simulink model "DAB"  (R2018b)
settings: Solver=ode23t  StartTime=0.0  StopTime=3  RelTol=1e-3
libraries: powerlib x22, simulink x1
settings Model: Creator=joshua  LastModifiedBy=joshua

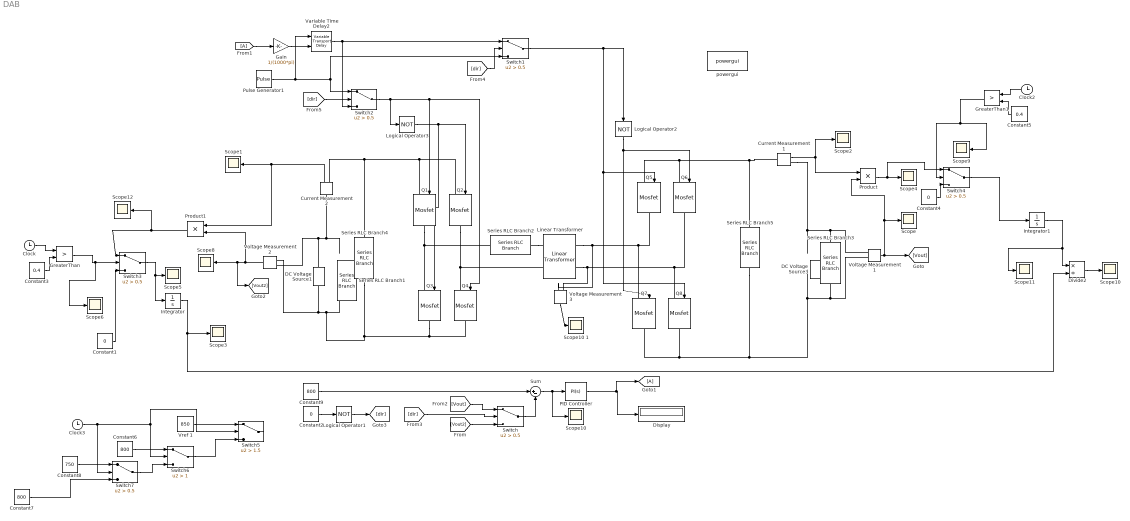
== system DAB ==
  Clock : Clock
  Clock2 : Clock
  Clock3 : Clock
  Constant1 : Constant  Value=0
  Constant2 : Constant  Value=0
  Constant3 : Constant  Value=0.4
  Constant4 : Constant  Value=0
  Constant5 : Constant  Value=0.4
  Constant6 : Constant  Value=800
  Constant7 : Constant  Value=800
  Constant8 : Constant  Value=750
  Constant9 : Constant  Value=800
  Current Measurement1 : powerlib/Measurements/Current Measurement  PhasorSimulation=off  OutputType=Complex  PSBequivalent=0
  Current Measurement2 : powerlib/Measurements/Current Measurement  PhasorSimulation=off  OutputType=Complex  PSBequivalent=0
  DC Voltage Source1 : powerlib/Electrical Sources/DC Voltage Source  Amplitude=800  Measurements=None
  DC Voltage Source3 : powerlib/Electrical Sources/DC Voltage Source  Amplitude=800  Measurements=None
  Display : Display
  Divide2 : Product  Inputs=*/
  Gain : Gain  Gain=1/(1000*pi)
  GreaterThan : RelationalOperator  Operator=>  OutDataTypeStr=boolean  RndMeth=Simplest
  GreaterThan1 : RelationalOperator  Operator=>  OutDataTypeStr=boolean  RndMeth=Simplest
  Integrator : Integrator
  Integrator1 : Integrator
  Linear Transformer : powerlib/Elements/Linear Transformer  UNITS=SI  NominalPower=[800 50000]  winding1=[5 0 0]  winding2=[5 0 0]  ThreeWindings=off  winding3=[3.15e+05 0.7938 0.084225]  RmLm=[1.0804e2 1e-3]  Measurements=None  DataType=on
  Logical Operator1 : Logic  Operator=NOT  Inputs=1  AllPortsSameDT=off  OutDataTypeStr=boolean
  Logical Operator2 : Logic  Operator=NOT  Inputs=1  AllPortsSameDT=off  OutDataTypeStr=boolean
  Logical Operator3 : Logic  Operator=NOT  Inputs=1  AllPortsSameDT=off  OutDataTypeStr=boolean
  PID Controller : simulink/Continuous/PID Controller  Controller=PI  Form=Parallel  TimeDomain=Continuous-time  SampleTime=-1  IntegratorMethod=Forward Euler  FilterMethod=Forward Euler  ControllerParametersSource=internal  P=0.001  I=0.025  D=0  UseFilter=on  N=100  TunerSelectOption=Transfer Function Based (PID Tuner App)  InitialConditionSource=internal  InitialConditionForIntegrator=0  InitialConditionForFilter=0  DifferentiatorICPrevScaledInput=0  ExternalReset=none  TrackingMode=off  Kt=1  LimitOutput=off  UpperSaturationLimit=0.5  LowerSaturationLimit=-0.5  LinearizeAsGain=on  AntiWindupMode=clamping  Kb=1  POutMin=[]  POutMax=[]  IOutMin=[]  IOutMax=[]  DOutMin=[]  DOutMax=[]  NOutMin=[]  NOutMax=[]  SumOutMin=[]  SumOutMax=[]  SaturationOutMin=[]  SaturationOutMax=[]  PParamMin=[]  PParamMax=[]  IParamMin=[]  IParamMax=[]  DParamMin=[]  DParamMax=[]  NParamMin=[]  NParamMax=[]  KbParamMin=[]  KbParamMax=[]  KtParamMin=[]  KtParamMax=[]  KbOutMin=[]  KbOutMax=[]  KtOutMin=[]  KtOutMax=[]  IntegratorOutMin=[]  IntegratorOutMax=[]  FilterOutMin=[]  FilterOutMax=[]  SumI1OutMin=[]  SumI1OutMax=[]  SumI2OutMin=[]  SumI2OutMax=[]  SumI3OutMin=[]  SumI3OutMax=[]  SumI4OutMin=[]  SumI4OutMax=[]  SumDOutMin=[]  SumDOutMax=[]  DifferentiatorOutMin=[]  DifferentiatorOutMax=[]  FilterDiffOutCoefMin=[]  FilterDiffOutCoefMax=[]  ReciprocalOutMin=[]  ReciprocalOutMax=[]  SumDenOutMin=[]  SumDenOutMax=[]  SumNumOutMin=[]  SumNumOutMax=[]  DivideOutMin=[]  DivideOutMax=[]  IntegratorContinuousStateAttributes=''  IntegratorStateMustResolveToSignalObject=off  IntegratorRTWStateStorageClass=Auto  FilterContinuousStateAttributes=''  FilterStateMustResolveToSignalObject=off  FilterRTWStateStorageClass=Auto  ParallelPVariant=InternalParameters  IdealPVariant=Disabled  IVariant=InternalParameters  DVariant=Disabled  IntegratorVariant=Continuous  SatVariant=Disabled  AWVariant=Passthrough  PCopyVariant=Disabled  TRVariant=Disabled  FdbkBlocksVariant=Forward  IdealPFdbkVariant=Disabled  SatFdbkVariant=Disabled  DerivativeFilterVariant=Disabled  NVariant=Disabled  NCopyVariant=Disabled_SignalSpec  FilterICVariant=Disabled  IntegratorICVariant=InternalICs  ExternalResetVariant=Disabled  TRSumVariant=Passthrough  SumFdbkVariant=Disabled  SumVariant=Sum_PI
  Product : Product
  Product1 : Product
  Pulse Generator1 : DiscretePulseGenerator  PulseType=Time based  Period=1/50000  PulseWidth=50
  Q{1..8} (8 alike) : powerlib/Power Electronics/Mosfet  Ron=0.1  Lon=0  Rd=0.01  Vfd=0  IC=0  Rs=1e5  Cs=inf  Measurements=off
  Scope{,1..6,8..12} (12 alike) : Scope
  "Scope10 " : Scope
  Scope10 1 : Scope
  Series RLC Branch1 : powerlib/Elements/Series RLC Branch  LConnTagsString=__new0  RConnTagsString=__new0  BranchType=R  Resistance=6.4  Inductance=1e-3  SetiL0=off  InitialCurrent=0  Capacitance=1e-6  Setx0=off  InitialVoltage=0  Measurements=None
  Series RLC Branch2 : powerlib/Elements/Series RLC Branch  LConnTagsString=__new0  RConnTagsString=__new0  BranchType=L  Resistance=1000  Inductance=1e-6  SetiL0=off  InitialCurrent=0  Capacitance=1e-6  Setx0=off  InitialVoltage=0  Measurements=None
  Series RLC Branch3 : powerlib/Elements/Series RLC Branch  LConnTagsString=__new0  RConnTagsString=__new0  BranchType=R  Resistance=64  Inductance=1e-3  SetiL0=off  InitialCurrent=0  Capacitance=1e-6  Setx0=off  InitialVoltage=0  Measurements=None
  Series RLC Branch4 : powerlib/Elements/Series RLC Branch  LConnTagsString=__new0  RConnTagsString=__new0  BranchType=RC  Resistance=0.0001  Inductance=1e-3  SetiL0=off  InitialCurrent=0  Capacitance=1000e-5  Setx0=off  InitialVoltage=0  Measurements=None
  Series RLC Branch5 : powerlib/Elements/Series RLC Branch  LConnTagsString=__new0  RConnTagsString=__new0  BranchType=RC  Resistance=0.0001  Inductance=1e-3  SetiL0=off  InitialCurrent=0  Capacitance=1000e-5  Setx0=off  InitialVoltage=0  Measurements=None
  Sum : Sum  Inputs=|+-
  Switch{,1..4,7} (6 alike) : Switch  Criteria=u2 > Threshold  Threshold=0.5
  Switch5 : Switch  Criteria=u2 > Threshold  Threshold=1.5
  Switch6 : Switch  Criteria=u2 > Threshold  Threshold=1
  Variable Time Delay2 : VariableTransportDelay  MaximumDelay=10
  Voltage Measurement1 : powerlib/Measurements/Voltage Measurement  PhasorSimulation=off  OutputType=Magnitude  PSBequivalent=0
  Voltage Measurement2 : powerlib/Measurements/Voltage Measurement  PhasorSimulation=off  OutputType=Magnitude  PSBequivalent=0
  Voltage Measurement3 : powerlib/Measurements/Voltage Measurement  PhasorSimulation=off  OutputType=Magnitude  PSBequivalent=0
  Vref 1 : Constant  Value=850
  powergui : powerlib/powergui  Priority=1  SimulationMode=Discrete  SampleTime=1e-7  frequency=60  Iterations=50  frequencyindice=0  Pbase=100e6  ErrMax=1e-4  UnitsV=kV  UnitsW=MW  buscounter=0  FunctionMessages=off  echomessages=off  EnableUseOfTLC=off  CurrentSourceSwitches=off  DisableSnubberDevices=off  DisableRonSwitches=off  DisableVfSwitches=off  DisplayEquations=off  SolverType=Tustin/Backward Euler (TBE)  Interpol=off  ExternalGateDelay=off  methode=off  Ts=100  x0status=blocks  SPID=on  SwTol=0  HookPort=off  RestoreLinks=warning  ResistiveCurrentMeasurement=off  Frange=[0:2:500]  Ylog=off  Xlog=on  ShowGrid=off  save=off  variable=ZData  structure=ScopeData  ZoomFFT=on  StartTime=0.5  cycles=20  DisplayStyle=1  fundamental=50000  FreqAxis=off  MaxFrequency=500000  frequencyindicesteady=1  RmsSteady=1  display=off
  wires:
  Voltage Measurement1/1 -> [Vout], Product/2, Scope/1
  Current Measurement1/1 -> Scope2/1, Product/1
  Sum/1 -> "Scope10 "/1, PID Controller/1
  Constant9/1 -> Sum/1
  PID Controller/1 -> [A], Display/1
  [A] -> Gain/1
  Voltage Measurement2/1 -> Product1/2, [Vout2], Scope8/1
  [Vout2] -> Switch/3
  [dir] -> Switch/2
  [dir] -> Switch1/2
  [Vout] -> Switch/1
  Switch/1 -> Sum/2
  Variable Time Delay2/1 -> Switch1/1, Switch2/3
  Pulse Generator1/1 -> Variable Time Delay2/1, Switch2/1, Switch1/3
  Voltage Measurement3/1 -> Scope10 1/1
  Switch1/1 -> Logical Operator2/1, Q8/1, Q5/1
  Switch2/1 -> Q4/1, Q1/1, Logical Operator3/1
  Logical Operator2/1 -> Q7/1, Q6/1
  Logical Operator3/1 -> Q2/1, Q3/1
  Constant2/1 -> Logical Operator1/1
  Logical Operator1/1 -> [dir]
  [dir] -> Switch2/2
  Gain/1 -> Variable Time Delay2/2
  Current Measurement2/1 -> Product1/1, Scope1/1
  Product/1 -> Switch4/1, Scope4/1
  Product1/1 -> Scope12/1, Switch3/1
  Constant1/1 -> Switch3/3
  Clock/1 -> GreaterThan/1
  Constant3/1 -> GreaterThan/2
  GreaterThan/1 -> Scope6/1, Switch3/2
  Switch3/1 -> Scope5/1, Integrator/1
  Constant4/1 -> Switch4/3
  Constant5/1 -> GreaterThan1/2
  Clock2/1 -> GreaterThan1/1
  GreaterThan1/1 -> Scope9/1, Switch4/2
  Divide2/1 -> Scope10/1
  Integrator/1 -> Scope3/1, Divide2/2
  Switch4/1 -> Integrator1/1
  Integrator1/1 -> Divide2/1, Scope11/1
  Constant6/1 -> Switch6/1
  Switch7/1 -> Switch6/3
  Constant7/1 -> Switch7/3
  Constant8/1 -> Switch7/1
  Switch6/1 -> Switch5/3
  Clock3/1 -> Switch6/2, Switch5/2, Switch7/2
  Vref 1/1 -> Switch5/1
  connections:
  Q4/LConn1 -- Linear Transformer/LConn2 -- Q2/RConn1
  Series RLC Branch2/RConn1 -- Q1/RConn1 -- Q3/LConn1
  Voltage Measurement1/LConn2 -- Series RLC Branch3/RConn1 -- Q8/RConn1 -- Q7/RConn1 -- Series RLC Branch5/RConn1
  Voltage Measurement1/LConn1 -- Series RLC Branch3/LConn1 -- Current Measurement1/RConn1
  Series RLC Branch2/LConn1 -- Linear Transformer/LConn1
  DC Voltage Source1/RConn1 -- Voltage Measurement2/LConn1 -- Current Measurement2/LConn1
  Linear Transformer/RConn1 -- Q5/RConn1 -- Q7/LConn1 -- Voltage Measurement3/LConn2
  Linear Transformer/RConn2 -- Q6/RConn1 -- Q8/LConn1 -- Voltage Measurement3/LConn1
  Series RLC Branch5/LConn1 -- Q6/LConn1 -- Q5/LConn1 -- Current Measurement1/LConn1
  Q2/LConn1 -- Series RLC Branch4/LConn1 -- Current Measurement2/RConn1 -- Q1/LConn1
  Voltage Measurement2/LConn2 -- DC Voltage Source1/LConn1 -- Series RLC Branch4/RConn1 -- Q3/RConn1 -- Q4/RConn1
